simulink model "IF"  (R2021b)
settings: Solver=FixedStepAuto  StartTime=0.0  StopTime=10.0  FixedStep=1e-4  RelTol=1e-3
undefined symbols (not defined in the file): curr_d_ki, curr_d_kp, curr_q_ki, curr_q_kp, CurrKi, CurrKp, DiscIntNeverNeededParam, Pn, Udc
libraries: slpidlib x2, mcbplantlib x1, autolibpmsmexterior x1
settings Model: DataDictionary=IF.sldd  Creator=Administrator  LastModifiedBy=fwdde
settings OptimizationCC: DefaultParameterBehavior=Inlined  UseDivisionForNetSlopeComputation=on  GainParamInheritBuiltInType=on  UseFloatMulNetSlope=on  InlineInvariantSignals=on  PassReuseOutputArgsAs=Individual arguments  ZeroExternalMemoryAtStartup=off  ZeroInternalMemoryAtStartup=off  NoFixptDivByZeroProtection=on  EfficientFloat2IntCast=on  LifeSpan=1  OptimizeBlockOrder=speed  DifferentSizesBufferReuse=on  EfficientTunableParamExpr=on
settings DebuggingCC: ParameterTunabilityLossMsg=error
settings HardwareCC: ProdBitPerPointer=32  ProdBitPerSizeT=32  ProdBitPerPtrDiffT=32  ProdLargestAtomicInteger=Long  ProdLargestAtomicFloat=Double  ProdWordSize=32  ProdLongLongMode=on  ProdHWDeviceType=ARM Compatible->ARM Cortex-M
settings SFSimCC: MATLABDynamicMemAlloc=off
settings RTWCC: Description=Embedded Coder  SystemTargetFile=ert.tlc  GenCodeOnly=on  TemplateMakefile=ert_default_tmf  GenerateReport=on  LaunchReport=on  GenerateCodeReplacementReport=on
settings CodeAppCC: ForceParamTrailComments=on  IgnoreCustomStorageClasses=off  OperatorAnnotations=on  SimulinkDataObjDesc=on  SFDataObjDesc=on  CustomSymbolStrGlobalVar=rt$N$M  CustomSymbolStrType=$N$M  CustomSymbolStrFcn=$N$M$F  CustomSymbolStrMacro=$N$M  InsertBlockDesc=on
settings ERTTargetCC: TargetLangStandard=C99 (ISO)  CodeReplacementLibrary=ARM Cortex-M  GenerateSampleERTMain=on  IncludeMdlTerminateFcn=off  CombineSignalStateStructs=on  SupportAbsoluteTime=off  SupportComplex=off  SupportNonInlinedSFcns=on  InlinedParameterPlacement=NonHierarchical  ERTCustomFileTemplate=example_file_process.tlc  ERTFilePackagingFormat=CompactWithDataFile

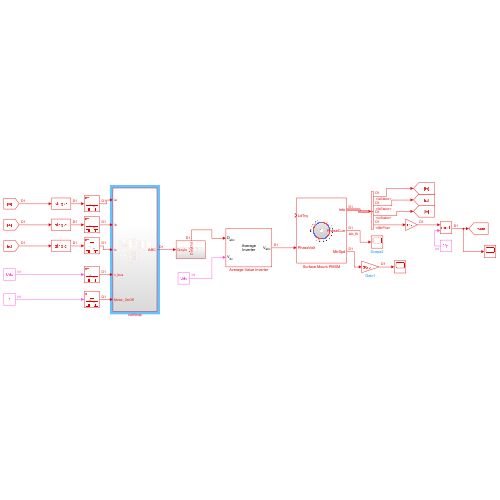
[thumbnail: Simulink's stored preview of the top-level diagram]
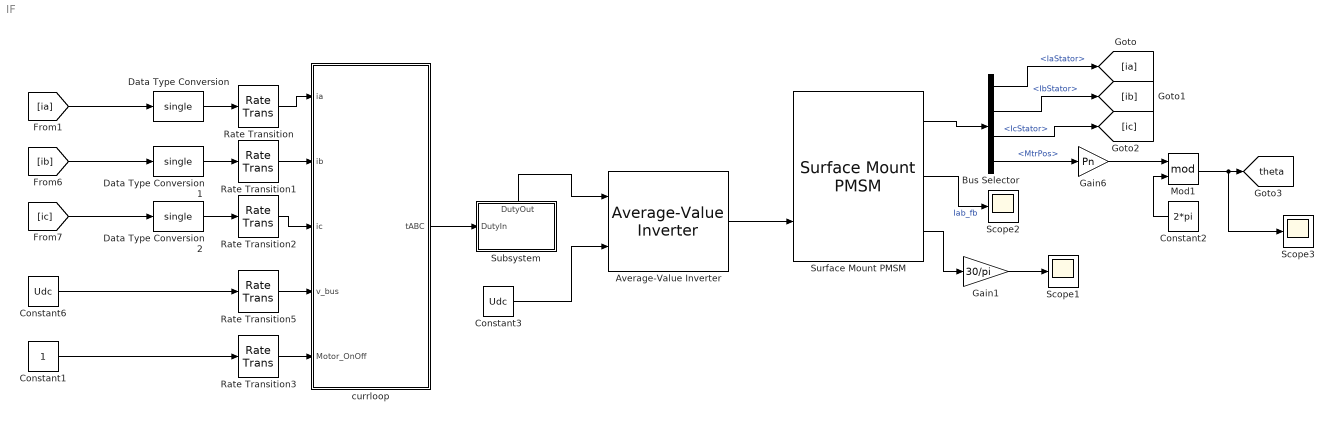
== system IF ==
  Average-Value Inverter : mcbplantlib/Average-Value Inverter
  Bus Selector : BusSelector  OutputSignals=IaStator,IbStator,IcStator,MtrPos
  Constant1 : Constant  OutDataTypeStr=single
  Constant2 : Constant  Value=2*pi  OutDataTypeStr=single
  Constant3 : Constant  Value=Udc
  Constant6 : Constant  Value=Udc  OutDataTypeStr=single
  Data Type Conversion : DataTypeConversion  OutDataTypeStr=single
  Data Type Conversion1 : DataTypeConversion  OutDataTypeStr=single
  Data Type Conversion2 : DataTypeConversion  OutDataTypeStr=single
  Gain1 : Gain  Gain=30/pi  OutDataTypeStr=single
  Gain6 : Gain  Gain=Pn  OutDataTypeStr=single
  Mod1 : Math  Operator=mod  OutputSignalType=real  SaturateOnIntegerOverflow=on
  Rate Transition{,1..3,5} (5 alike) : RateTransition
  Scope1 : Scope
  Scope2 : Scope
  Scope3 : Scope
  Subsystem : Subsystem
      settings: PortSchema="{\"entries\":[{\"content\":{\"sides\":[{\"content\":{\"connectorIds\":[\"In1\"]},\"type\":\"ConnectorPlacement.EquallySpacedRectSide\",\"uuid\":\"8ccc51de-fa2a-4900-80a3-4cdf9aa76f01\"},{\"content\":{\"connectorIds\":[],\"side\":\"RIGHT\"},\"type\":\"ConnectorPlacement.EquallySpacedRectSide\",\"uuid\":\"32c06e0d-3f1d-4948-af96-e310e54308a0\"},{\"content\":{\"connectorIds\":[\"Out1\"],\"side\":\"TOP\"},\"type\":\"ConnectorPlacement.EquallySpacedRectSide\",\"uuid\":\"a9066067-2c54-42a8-b4d7-fb86ac71b860\"}]},\"type\":\"ConnectorPlacement.EquallySpacedConnector\",\"uuid\":\"e4576975-acad-4e16-822f-2c2e7f23d7a7\"}],\"packageUris\":[\"http://schema.mathworks.com/mf0/Connector/R2020b\"],\"version\":\"1.0\"}"
  Surface Mount PMSM : autolibpmsmexterior/Surface Mount PMSM  port_config=Torque  sim_type=Discrete  Ts=1e-4  P=Pn  Rs=Rs  Ldq_=L  KConstText=Permanent flux linkage constant (lambda_pm):  lambda_pm=flux  Ke=0.0059268  Kt=0.061  mechanical=[75e-6, 8e-5, 0]  idq0=[0 0]  theta_init=4/5  omega_init=0  KConst=flux  lambda_pm_calc=flux  RefBlkName='autolibpmsmexterior/Surface Mount PMSM'  aMode=5  Ldq="[0.0017      0.0017]"
      settings: SourceProductBaseCode=PW,DR,MT,UV,VE
  currloop : Subsystem
  tag scope: theta=global
  wires:
  Constant3/1 -> Average-Value Inverter/2
  Subsystem/1(DutyOut) -> Average-Value Inverter/1
  Average-Value Inverter/1 -> Surface Mount PMSM/2
  Surface Mount PMSM/3 -> Gain1/1
  Bus Selector/1 -> [ia]  "<IaStator>"
  Bus Selector/2 -> [ib]  "<IbStator>"
  Bus Selector/3 -> [ic]  "<IcStator>"
  Surface Mount PMSM/1 -> Bus Selector/1
  [ia] -> Data Type Conversion/1
  [ic] -> Data Type Conversion2/1
  [ib] -> Data Type Conversion1/1
  Data Type Conversion/1 -> Rate Transition/1
  Data Type Conversion1/1 -> Rate Transition1/1
  Data Type Conversion2/1 -> Rate Transition2/1
  Constant6/1 -> Rate Transition5/1
  Surface Mount PMSM/2 -> Scope2/1  "Iab_fb"
  Gain6/1 -> Mod1/1
  Constant2/1 -> Mod1/2
  Bus Selector/4 -> Gain6/1  "<MtrPos>"
  Mod1/1 -> Scope3/1, [theta]
  Rate Transition/1 -> currloop/1(ia)
  Rate Transition1/1 -> currloop/2(ib)
  Rate Transition2/1 -> currloop/3(ic)
  Rate Transition5/1 -> currloop/4(v_bus)
  currloop/1(tABC) -> Subsystem/1(DutyIn)
  Rate Transition3/1 -> currloop/5(Motor_OnOff)
  Constant1/1 -> Rate Transition3/1
  Gain1/1 -> Scope1/1

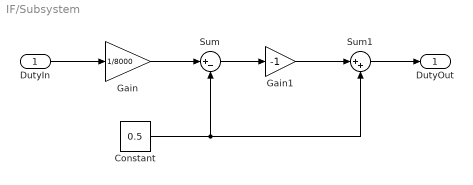
== system IF/Subsystem ==
  DutyIn : Inport
  Constant : Constant  Value=0.5  SampleTime=-1
  Gain : Gain  Gain=1/8000  ParamDataTypeStr=single
  Gain1 : Gain  Gain=-1
  Sum : Sum  Inputs=|+-
  Sum1 : Sum  Inputs=|++
  DutyOut : Outport
  wires:
  Sum/1 -> Gain1/1
  Constant/1 -> Sum1/2, Sum/2
  DutyIn/1 -> Gain/1
  Gain1/1 -> Sum1/1
  Sum1/1 -> DutyOut/1
  Gain/1 -> Sum/1

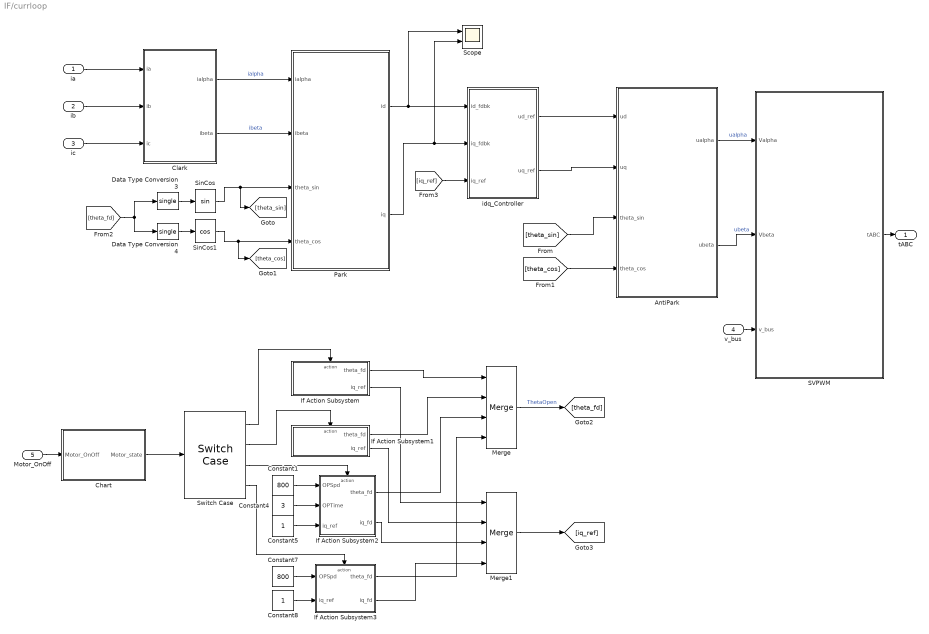
== system IF/currloop ==
  ia : Inport
  ib : Inport  Port=2
  ic : Inport  Port=3
  v_bus : Inport  Port=4
  Motor_OnOff : Inport  Port=5
  AntiPark : Subsystem
  Chart : Stateflow chart  TreatAsAtomicUnit=on
  Clark : Subsystem
  Constant1 : Constant  Value=800  OutDataTypeStr=single
  Constant4 : Constant  Value=3  OutDataTypeStr=single
  Constant5 : Constant  OutDataTypeStr=single
  Constant7 : Constant  Value=800  OutDataTypeStr=single
  Constant8 : Constant  OutDataTypeStr=single
  Data Type Conversion3 : DataTypeConversion  OutDataTypeStr=single
  Data Type Conversion4 : DataTypeConversion  OutDataTypeStr=single
  If Action Subsystem : Subsystem  TreatAsAtomicUnit=on
  If Action Subsystem1 : Subsystem  TreatAsAtomicUnit=on
  If Action Subsystem2 : Subsystem  TreatAsAtomicUnit=on
  If Action Subsystem3 : Subsystem  TreatAsAtomicUnit=on
  Merge : Merge  Inputs=4
  Merge1 : Merge  Inputs=4
  Park : Subsystem
  SVPWM : Subsystem  TreatAsAtomicUnit=on
  Scope : Scope  NumInputPorts=2
  SinCos : Trigonometry
  SinCos1 : Trigonometry  Operator=cos
  Switch Case : SwitchCase  CaseConditions={1,2,3,4}  ShowDefaultCase=off
  idq_Controller : Subsystem
  tABC : Outport
  wires:
  Data Type Conversion4/1 -> SinCos1/1
  Data Type Conversion3/1 -> SinCos/1
  AntiPark/2(ubeta) -> SVPWM/2(Vbeta)  "ubeta"
  AntiPark/1(ualpha) -> SVPWM/1(Valpha)  "ualpha"
  [theta_cos] -> AntiPark/4(theta_cos)
  [theta_sin] -> AntiPark/3(theta_sin)
  SinCos/1 -> Park/3(theta_sin), [theta_sin]
  [theta_fd] -> Data Type Conversion3/1, Data Type Conversion4/1
  SinCos1/1 -> Park/4(theta_cos), [theta_cos]
  v_bus/1 -> SVPWM/3(v_bus)
  SVPWM/1(tABC) -> tABC/1
  ib/1 -> Clark/2(ib)
  ia/1 -> Clark/1(ia)
  ic/1 -> Clark/3(ic)
  Clark/1(ialpha) -> Park/1(ialpha)  "ialpha"
  Clark/2(ibeta) -> Park/2(ibeta)  "ibeta"
  idq_Controller/1(ud_ref) -> AntiPark/1(ud)
  idq_Controller/2(uq_ref) -> AntiPark/2(uq)
  Park/1(id) -> Scope/1, idq_Controller/1(id_fdbk)
  Park/2(iq) -> Scope/2, idq_Controller/2(iq_fdbk)
  [iq_ref] -> idq_Controller/3(iq_ref)
  Constant1/1 -> If Action Subsystem2/1(OPSpd)
  Constant8/1 -> If Action Subsystem3/2(iq_ref)
  Switch Case/2 -> If Action Subsystem1/Action
  Chart/1(Motor_state) -> Switch Case/1
  Constant7/1 -> If Action Subsystem3/1(OPSpd)
  Switch Case/4 -> If Action Subsystem3/Action
  Constant4/1 -> If Action Subsystem2/2(OPTime)
  Constant5/1 -> If Action Subsystem2/3(iq_ref)
  Switch Case/1 -> If Action Subsystem/Action
  Switch Case/3 -> If Action Subsystem2/Action
  If Action Subsystem/1(theta_fd) -> Merge/1
  If Action Subsystem1/1(theta_fd) -> Merge/2
  If Action Subsystem2/1(theta_fd) -> Merge/3
  If Action Subsystem3/1(theta_fd) -> Merge/4
  If Action Subsystem/2(iq_ref) -> Merge1/1
  If Action Subsystem1/2(iq_ref) -> Merge1/2
  If Action Subsystem2/2(iq_fd) -> Merge1/3
  If Action Subsystem3/2(iq_fd) -> Merge1/4
  Merge/1 -> [theta_fd]  "ThetaOpen"
  Merge1/1 -> [iq_ref]
  Motor_OnOff/1 -> Chart/1(Motor_OnOff)

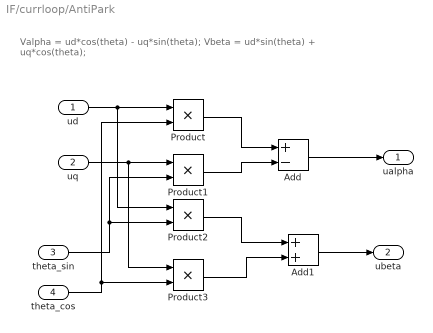
== system IF/currloop/AntiPark ==
  note: Valpha = ud*cos(theta) - uq*sin(theta);
      | Vbeta = ud*sin(theta) + uq*cos(theta);
  ud : Inport
  uq : Inport  Port=2
  theta_sin : Inport  Port=3
  theta_cos : Inport  Port=4
  Add : Sum  Inputs=+-
  Add1 : Sum
  Product{,1..3} (4 alike) : Product
  ualpha : Outport  OutDataTypeStr=single
  ubeta : Outport  Port=2  OutDataTypeStr=single
  wires:
  Product2/1 -> Add1/1
  Product/1 -> Add/1
  Add/1 -> ualpha/1
  Product3/1 -> Add1/2
  ud/1 -> Product/1, Product2/1
  theta_sin/1 -> Product1/2, Product2/2
  theta_cos/1 -> Product3/2, Product/2
  uq/1 -> Product1/1, Product3/1
  Product1/1 -> Add/2
  Add1/1 -> ubeta/1

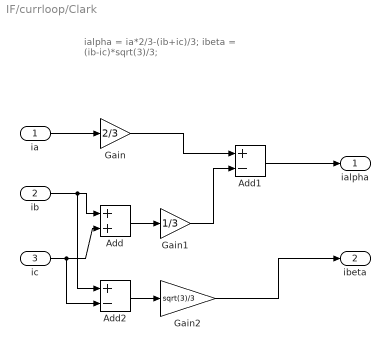
== system IF/currloop/Clark ==
  note: ialpha = ia*2/3-(ib+ic)/3;
      | ibeta = (ib-ic)*sqrt(3)/3;
  ia : Inport  OutDataTypeStr=single
  ib : Inport  Port=2  OutDataTypeStr=single
  ic : Inport  Port=3  OutDataTypeStr=single
  Add : Sum  AccumDataTypeStr=single  OutDataTypeStr=single
  Add1 : Sum  Inputs=+-  AccumDataTypeStr=single  OutDataTypeStr=single
  Add2 : Sum  Inputs=+-  AccumDataTypeStr=single  OutDataTypeStr=single
  Gain : Gain  Gain=2/3  ParamDataTypeStr=single
  Gain1 : Gain  Gain=1/3  ParamDataTypeStr=single
  Gain2 : Gain  Gain=sqrt(3)/3  ParamDataTypeStr=single
  ialpha : Outport  OutDataTypeStr=single
  ibeta : Outport  Port=2  OutDataTypeStr=single
  wires:
  Add1/1 -> ialpha/1
  ia/1 -> Gain/1
  Gain2/1 -> ibeta/1
  ib/1 -> Add/1, Add2/1
  Gain/1 -> Add1/1
  Add2/1 -> Gain2/1
  Add/1 -> Gain1/1
  ic/1 -> Add/2, Add2/2
  Gain1/1 -> Add1/2

== system IF/currloop/If Action Subsystem ==
  Action Port : ActionPort  ActionPortLabel=case [ 1 ]:
  Constant : Constant  Value=0  OutDataTypeStr=single
  Constant1 : Constant  Value=0  OutDataTypeStr=single
  theta_fd : Outport
  iq_ref : Outport  Port=2
  wires:
  Constant1/1 -> iq_ref/1
  Constant/1 -> theta_fd/1

== system IF/currloop/If Action Subsystem1 ==
  Action Port : ActionPort  ActionPortLabel=case [ 2 ]:
  Constant : Constant  Value=0  OutDataTypeStr=single
  Constant1 : Constant  Value=2  OutDataTypeStr=single
  theta_fd : Outport
  iq_ref : Outport  Port=2
  wires:
  Constant1/1 -> iq_ref/1
  Constant/1 -> theta_fd/1

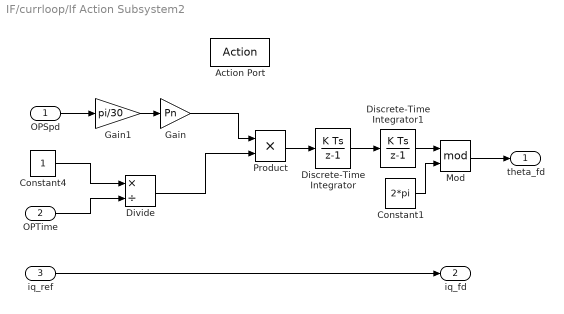
== system IF/currloop/If Action Subsystem2 ==
  OPSpd : Inport  OutDataTypeStr=single  PortDimensions=1
  OPTime : Inport  Port=2  OutDataTypeStr=single  PortDimensions=1
  iq_ref : Inport  Port=3
  Action Port : ActionPort  ActionPortLabel=case [ 3 ]:
  Constant1 : Constant  Value=2*pi  OutDataTypeStr=single
  Constant4 : Constant  OutDataTypeStr=single
  Discrete-Time Integrator : DiscreteIntegrator  SampleTime=-1  ICPrevOutput=DiscIntNeverNeededParam  ICPrevScaledInput=DiscIntNeverNeededParam
  Discrete-Time Integrator1 : DiscreteIntegrator  SampleTime=-1  ICPrevOutput=DiscIntNeverNeededParam  ICPrevScaledInput=DiscIntNeverNeededParam
  Divide : Product  Inputs=*/  OutDataTypeStr=single
  Gain : Gain  Gain=Pn
  Gain1 : Gain  Gain=pi/30  OutDataTypeStr=single
  Mod : Math  Operator=mod  SaturateOnIntegerOverflow=on
  Product : Product  OutDataTypeStr=single
  theta_fd : Outport
  iq_fd : Outport  Port=2
  wires:
  iq_ref/1 -> iq_fd/1
  Constant4/1 -> Divide/1
  Constant1/1 -> Mod/2
  Discrete-Time Integrator1/1 -> Mod/1
  Gain1/1 -> Gain/1
  Divide/1 -> Product/2
  Discrete-Time Integrator/1 -> Discrete-Time Integrator1/1
  Mod/1 -> theta_fd/1
  Gain/1 -> Product/1
  Product/1 -> Discrete-Time Integrator/1
  OPSpd/1 -> Gain1/1
  OPTime/1 -> Divide/2

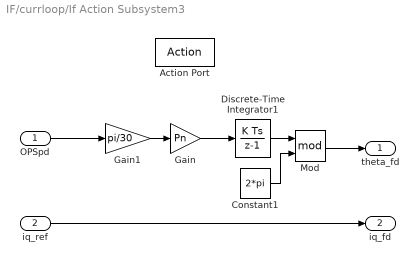
== system IF/currloop/If Action Subsystem3 ==
  OPSpd : Inport  OutDataTypeStr=single  PortDimensions=1
  iq_ref : Inport  Port=2
  Action Port : ActionPort  ActionPortLabel=case [ 4 ]:
  Constant1 : Constant  Value=2*pi  OutDataTypeStr=single
  Discrete-Time Integrator1 : DiscreteIntegrator  SampleTime=-1  ICPrevOutput=DiscIntNeverNeededParam  ICPrevScaledInput=DiscIntNeverNeededParam
  Gain : Gain  Gain=Pn
  Gain1 : Gain  Gain=pi/30  OutDataTypeStr=single
  Mod : Math  Operator=mod  SaturateOnIntegerOverflow=on
  theta_fd : Outport
  iq_fd : Outport  Port=2
  wires:
  iq_ref/1 -> iq_fd/1
  OPSpd/1 -> Gain1/1
  Discrete-Time Integrator1/1 -> Mod/1
  Constant1/1 -> Mod/2
  Gain/1 -> Discrete-Time Integrator1/1
  Gain1/1 -> Gain/1
  Mod/1 -> theta_fd/1

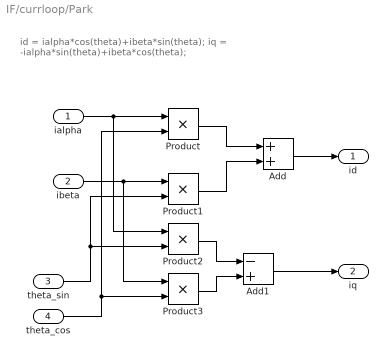
== system IF/currloop/Park ==
  note: id = ialpha*cos(theta)+ibeta*sin(theta);
      | iq = -ialpha*sin(theta)+ibeta*cos(theta);
  ialpha : Inport  OutDataTypeStr=single
  ibeta : Inport  Port=2  OutDataTypeStr=single
  theta_sin : Inport  Port=3  OutDataTypeStr=single
  theta_cos : Inport  Port=4  OutDataTypeStr=single
  Add : Sum  AccumDataTypeStr=single  OutDataTypeStr=single
  Add1 : Sum  Inputs=-+  AccumDataTypeStr=single  OutDataTypeStr=single
  Product{,1..3} (4 alike) : Product  OutDataTypeStr=single
  id : Outport  OutDataTypeStr=single
  iq : Outport  Port=2  OutDataTypeStr=single
  wires:
  theta_cos/1 -> Product/2, Product3/2
  ibeta/1 -> Product1/1, Product3/1
  Product1/1 -> Add/2
  Add1/1 -> iq/1
  Add/1 -> id/1
  Product3/1 -> Add1/2
  ialpha/1 -> Product/1, Product2/1
  Product2/1 -> Add1/1
  Product/1 -> Add/1
  theta_sin/1 -> Product1/2, Product2/2

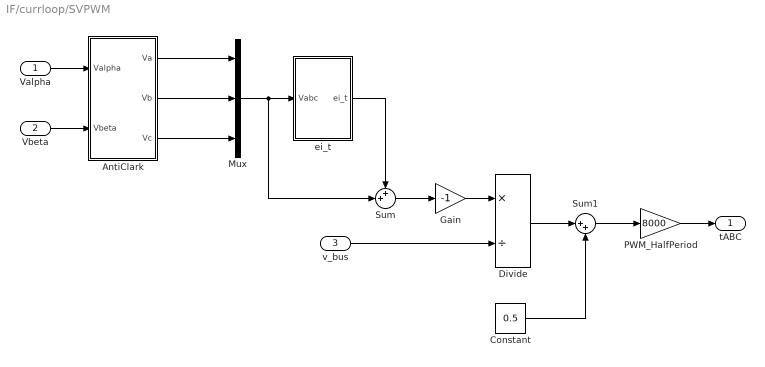
== system IF/currloop/SVPWM ==
  Valpha : Inport  OutDataTypeStr=single
  Vbeta : Inport  Port=2  OutDataTypeStr=single
  v_bus : Inport  Port=3  OutDataTypeStr=single
  AntiClark : Subsystem
  Constant : Constant  Value=0.5  OutDataTypeStr=single
  Divide : Product  Inputs=*/  OutDataTypeStr=single
  Gain : Gain  Gain=-1  OutDataTypeStr=single
  Mux : Mux  Inputs=3
  PWM_HalfPeriod : Gain  Gain=8000  OutDataTypeStr=single
  Sum : Sum  Inputs=++|  OutDataTypeStr=single
  Sum1 : Sum  Inputs=|++  OutDataTypeStr=single
  ei_t : Subsystem
  tABC : Outport  OutDataTypeStr=single
  wires:
  Gain/1 -> Divide/1
  v_bus/1 -> Divide/2
  PWM_HalfPeriod/1 -> tABC/1
  Sum1/1 -> PWM_HalfPeriod/1
  Constant/1 -> Sum1/2
  Divide/1 -> Sum1/1
  Mux/1 -> ei_t/1(Vabc), Sum/2
  Sum/1 -> Gain/1
  AntiClark/3(Vc) -> Mux/3
  AntiClark/2(Vb) -> Mux/2
  AntiClark/1(Va) -> Mux/1
  ei_t/1(ei_t) -> Sum/1
  Vbeta/1 -> AntiClark/2(Vbeta)
  Valpha/1 -> AntiClark/1(Valpha)

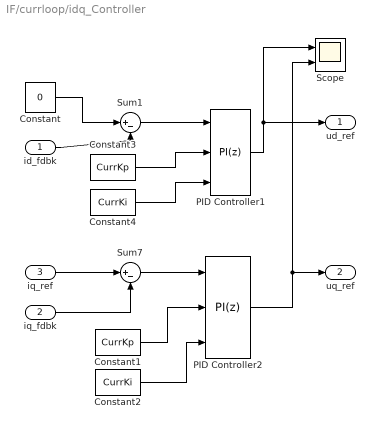
== system IF/currloop/idq_Controller ==
  id_fdbk : Inport  OutDataTypeStr=single
  iq_fdbk : Inport  Port=2  OutDataTypeStr=single
  iq_ref : Inport  Port=3  OutDataTypeStr=single
  Constant : Constant  Value=0  OutDataTypeStr=single
  Constant1 : Constant  Value=CurrKp  OutDataTypeStr=single
  Constant2 : Constant  Value=CurrKi  OutDataTypeStr=single
  Constant3 : Constant  Value=CurrKp  OutDataTypeStr=single
  Constant4 : Constant  Value=CurrKi  OutDataTypeStr=single
  PID Controller1 : slpidlib/PID Controller  Controller=PI  Form=Parallel  TimeDomain=Discrete-time  UseExternalTs=off  SampleTime=-1  IntegratorMethod=Forward Euler  FilterMethod=Forward Euler  ControllerParametersSource=external  P=curr_d_kp  I=curr_d_ki  D=0  UseFilter=on  N=100  TunerSelectOption=Transfer Function Based (PID Tuner App)  InitialConditionSource=internal  InitialConditionForIntegrator=0  InitialConditionForFilter=0  DifferentiatorICPrevScaledInput=0  ExternalReset=none  TrackingMode=off  Kt=1  LimitOutput=on  SatLimitsSource=internal  UpperSaturationLimit=24*0.9/sqrt(3)  LowerSaturationLimit=-24*0.9/sqrt(3)  LinearizeAsGain=on  AntiWindupMode=clamping  Kb=1  PGainOutDataTypeStr=single  PProdOutDataTypeStr=single  POutMin=[]  POutMax=[]  IGainOutDataTypeStr=int16  IProdOutDataTypeStr=int16  IOutMin=[]  IOutMax=[]  DOutMin=[]  DOutMax=[]  NOutMin=[]  NOutMax=[]  SumOutDataTypeStr=single  SumOutMin=[]  SumOutMax=[]  SaturationOutDataTypeStr=single  SaturationOutMin=[]  SaturationOutMax=[]  PParamMin=[]  PParamMax=[]  IParamMin=[]  IParamMax=[]  DParamMin=[]  DParamMax=[]  NParamMin=[]  NParamMax=[]  KbParamMin=[]  KbParamMax=[]  KtParamMin=[]  KtParamMax=[]  KbOutMin=[]  KbOutMax=[]  KtOutMin=[]  KtOutMax=[]  IntegratorOutMin=[]  IntegratorOutMax=[]  FilterOutMin=[]  FilterOutMax=[]  SumI1OutMin=[]  SumI1OutMax=[]  SumI2OutMin=[]  SumI2OutMax=[]  SumI3OutMin=[]  SumI3OutMax=[]  SumI4OutMin=[]  SumI4OutMax=[]  SumDOutMin=[]  SumDOutMax=[]  DifferentiatorOutMin=[]  DifferentiatorOutMax=[]  FilterDiffOutCoefMin=[]  FilterDiffOutCoefMax=[]  ReciprocalOutMin=[]  ReciprocalOutMax=[]  SumDenOutMin=[]  SumDenOutMax=[]  SumNumOutMin=[]  SumNumOutMax=[]  DivideOutMin=[]  DivideOutMax=[]  UdiffTsProdOutMin=[]  UdiffTsProdOutMax=[]  NTsProdOutMin=[]  NTsProdOutMax=[]  UintegralTsProdOutMin=[]  UintegralTsProdOutMax=[]  UngainTsProdOutMin=[]  UngainTsProdOutMax=[]  IntegratorContinuousStateAttributes=''  IntegratorStateMustResolveToSignalObject=off  IntegratorRTWStateStorageClass=Auto  FilterContinuousStateAttributes=''  FilterStateMustResolveToSignalObject=off  FilterRTWStateStorageClass=Auto  ParallelPVariant=ExternalParameters  IdealPVariant=Disabled  IVariant=ExternalParameters  DVariant=Disabled  IntegratorVariant=Discrete  SatVariant=Enabled  AWVariant=DiscClampingParallel  PCopyVariant=Disabled  TRVariant=Disabled  FdbkBlocksVariant=Forward  IdealPFdbkVariant=Disabled  SatFdbkVariant=Disabled  DerivativeFilterVariant=Disabled  NVariant=Disabled  NCopyVariant=Disabled_SignalSpec  FilterICVariant=Disabled  IntegratorICVariant=InternalICs  ExternalResetVariant=Disabled  TRSumVariant=Passthrough  SumFdbkVariant=Disabled  SumVariant=Sum_PI  TsampFilterVariant=InternalTs  TsampNgainVariant=Passthrough  TsampIntegralVariant=Passthrough  ExternalSaturationOutDataTypeStr=Inherit: Same as second input
  PID Controller2 : slpidlib/PID Controller  Controller=PI  Form=Parallel  TimeDomain=Discrete-time  UseExternalTs=off  SampleTime=-1  IntegratorMethod=Forward Euler  FilterMethod=Forward Euler  ControllerParametersSource=external  P=curr_q_kp  I=curr_q_ki  D=0  UseFilter=on  N=100  TunerSelectOption=Transfer Function Based (PID Tuner App)  InitialConditionSource=internal  InitialConditionForIntegrator=0  InitialConditionForFilter=0  DifferentiatorICPrevScaledInput=0  ExternalReset=none  TrackingMode=off  Kt=1  LimitOutput=on  SatLimitsSource=internal  UpperSaturationLimit=24*0.9/sqrt(3)  LowerSaturationLimit=-24*0.9/sqrt(3)  LinearizeAsGain=on  AntiWindupMode=clamping  Kb=1  PGainOutDataTypeStr=single  PProdOutDataTypeStr=single  POutMin=[]  POutMax=[]  IGainOutDataTypeStr=single  IProdOutDataTypeStr=single  IOutMin=[]  IOutMax=[]  DOutMin=[]  DOutMax=[]  NOutMin=[]  NOutMax=[]  SumOutDataTypeStr=single  SumOutMin=[]  SumOutMax=[]  SaturationOutDataTypeStr=single  SaturationOutMin=[]  SaturationOutMax=[]  PParamMin=[]  PParamMax=[]  IParamMin=[]  IParamMax=[]  DParamMin=[]  DParamMax=[]  NParamMin=[]  NParamMax=[]  KbParamMin=[]  KbParamMax=[]  KtParamMin=[]  KtParamMax=[]  KbOutMin=[]  KbOutMax=[]  KtOutMin=[]  KtOutMax=[]  IntegratorOutMin=[]  IntegratorOutMax=[]  FilterOutMin=[]  FilterOutMax=[]  SumI1OutMin=[]  SumI1OutMax=[]  SumI2OutMin=[]  SumI2OutMax=[]  SumI3OutMin=[]  SumI3OutMax=[]  SumI4OutMin=[]  SumI4OutMax=[]  SumDOutMin=[]  SumDOutMax=[]  DifferentiatorOutMin=[]  DifferentiatorOutMax=[]  FilterDiffOutCoefMin=[]  FilterDiffOutCoefMax=[]  ReciprocalOutMin=[]  ReciprocalOutMax=[]  SumDenOutMin=[]  SumDenOutMax=[]  SumNumOutMin=[]  SumNumOutMax=[]  DivideOutMin=[]  DivideOutMax=[]  UdiffTsProdOutMin=[]  UdiffTsProdOutMax=[]  NTsProdOutMin=[]  NTsProdOutMax=[]  UintegralTsProdOutMin=[]  UintegralTsProdOutMax=[]  UngainTsProdOutMin=[]  UngainTsProdOutMax=[]  IntegratorContinuousStateAttributes=''  IntegratorStateMustResolveToSignalObject=off  IntegratorRTWStateStorageClass=Auto  FilterContinuousStateAttributes=''  FilterStateMustResolveToSignalObject=off  FilterRTWStateStorageClass=Auto  ParallelPVariant=ExternalParameters  IdealPVariant=Disabled  IVariant=ExternalParameters  DVariant=Disabled  IntegratorVariant=Discrete  SatVariant=Enabled  AWVariant=DiscClampingParallel  PCopyVariant=Disabled  TRVariant=Disabled  FdbkBlocksVariant=Forward  IdealPFdbkVariant=Disabled  SatFdbkVariant=Disabled  DerivativeFilterVariant=Disabled  NVariant=Disabled  NCopyVariant=Disabled_SignalSpec  FilterICVariant=Disabled  IntegratorICVariant=InternalICs  ExternalResetVariant=Disabled  TRSumVariant=Passthrough  SumFdbkVariant=Disabled  SumVariant=Sum_PI  TsampFilterVariant=InternalTs  TsampNgainVariant=Passthrough  TsampIntegralVariant=Passthrough  ExternalSaturationOutDataTypeStr=Inherit: Same as second input
  Scope : Scope  NumInputPorts=2
  Sum1 : Sum  Inputs=|+-  AccumDataTypeStr=single  OutDataTypeStr=single
  Sum7 : Sum  Inputs=|+-  AccumDataTypeStr=single  OutDataTypeStr=single
  ud_ref : Outport  OutDataTypeStr=single
  uq_ref : Outport  Port=2  OutDataTypeStr=single
  wires:
  id_fdbk/1 -> Sum1/2
  Constant/1 -> Sum1/1
  iq_fdbk/1 -> Sum7/2
  Sum1/1 -> PID Controller1/1
  Sum7/1 -> PID Controller2/1
  PID Controller1/1 -> Scope/1, ud_ref/1
  PID Controller2/1 -> Scope/2, uq_ref/1
  iq_ref/1 -> Sum7/1
  Constant3/1 -> PID Controller1/2
  Constant4/1 -> PID Controller1/3
  Constant1/1 -> PID Controller2/2
  Constant2/1 -> PID Controller2/3

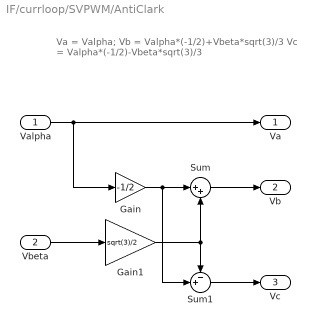
== system IF/currloop/SVPWM/AntiClark ==
  note: Va = Valpha;
      | Vb = Valpha*(-1/2)+Vbeta*sqrt(3)/3
      | Vc = Valpha*(-1/2)-Vbeta*sqrt(3)/3
  Valpha : Inport  OutDataTypeStr=single
  Vbeta : Inport  Port=2  OutDataTypeStr=single
  Gain : Gain  Gain=-1/2  OutDataTypeStr=single
  Gain1 : Gain  Gain=sqrt(3)/2  OutDataTypeStr=single
  Sum : Sum  Inputs=|++  OutDataTypeStr=single
  Sum1 : Sum  Inputs=-+|  OutDataTypeStr=single
  Va : Outport  OutDataTypeStr=single
  Vb : Outport  Port=2  OutDataTypeStr=single
  Vc : Outport  Port=3  OutDataTypeStr=single
  wires:
  Sum1/1 -> Vc/1
  Gain1/1 -> Sum1/1, Sum/2
  Sum/1 -> Vb/1
  Gain/1 -> Sum/1, Sum1/2
  Vbeta/1 -> Gain1/1
  Valpha/1 -> Va/1, Gain/1

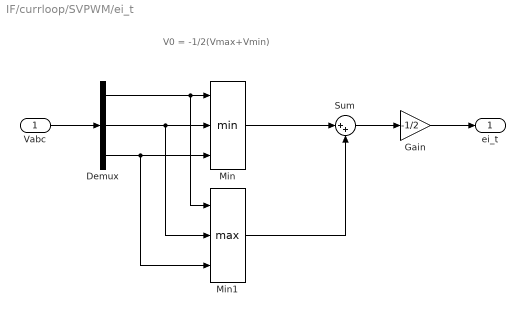
== system IF/currloop/SVPWM/ei_t ==
  note: V0 = -1/2(Vmax+Vmin)
  Vabc : Inport  OutDataTypeStr=single
  Demux : Demux  Outputs=3
  Gain : Gain  Gain=-1/2  OutDataTypeStr=single
  Min : MinMax  Inputs=3  OutDataTypeStr=single
  Min1 : MinMax  Function=max  Inputs=3  OutDataTypeStr=single
  Sum : Sum  Inputs=|++  OutDataTypeStr=single
  ei_t : Outport  OutDataTypeStr=single
  wires:
  Demux/3 -> Min/3, Min1/3
  Demux/2 -> Min1/2, Min/2
  Demux/1 -> Min/1, Min1/1
  Vabc/1 -> Demux/1
  Gain/1 -> ei_t/1
  Min1/1 -> Sum/2
  Sum/1 -> Gain/1
  Min/1 -> Sum/1

== stateflow chart IF/currloop/Chart ==
  state RunStage
    en:
    du:
    Motor_state = 4;
  state OpenStage
    en:
    du:
    Motor_state = 3;
  state AlignStage
    en:
    du:
    Motor_state = 2;
  state IDLE
    en:
    du:
    Motor_state = 1;
  (default) -> IDLE
  IDLE -> AlignStage : [Motor_OnOff ==1]
  AlignStage -> OpenStage [order 1] : [after(1000,tick)]
  OpenStage -> RunStage [order 2] : [after(30000,tick) ]
  AlignStage -> IDLE [order 2] : [Motor_OnOff == 0]
  OpenStage -> IDLE [order 1] : [Motor_OnOff ==0]
  RunStage -> IDLE : [Motor_OnOff ==0]
  data: Motor_OnOff input; Motor_state output
